simulink model "flyball"  (R2016b)
settings: Solver=VariableStepAuto  StartTime=0.0  StopTime=30  MaxStep=0.001  RelTol=1e-3
values from neighbouring files (symbols this model uses):
  g = 9.81    [simulateflyball.m]
  L = 0.2    [simulateflyball.m]
  M = 0.1    [simulateflyball.m]
  m = 0.2    [simulateflyball.m]
  thetaDotInitial = 0    [simulateflyball.m]
  thetaInitial = 0.0001    [simulateflyball.m]
  w = 6*pi    (= 18.8495559215)    [simulateflyball.m]
settings Model: Creator=kargto  LastModifiedBy=kargto

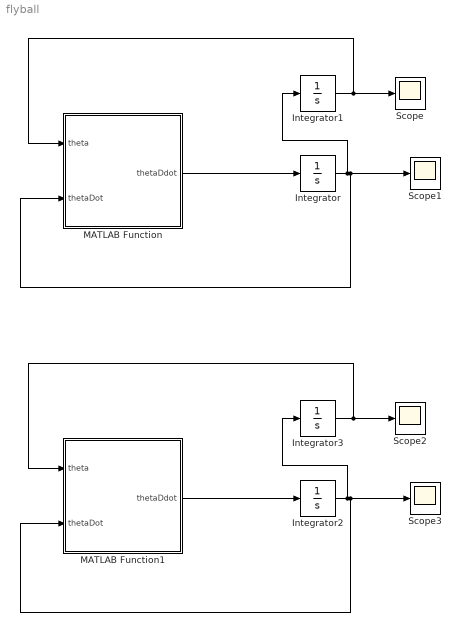
== system flyball ==
  Integrator : Integrator  InitialCondition=thetaDotInitial
  Integrator1 : Integrator  InitialCondition=thetaInitial
  Integrator2 : Integrator  InitialCondition=thetaDotInitial
  Integrator3 : Integrator  InitialCondition=thetaInitial
  MATLAB Function : MATLAB Function  TreatAsAtomicUnit=on
  MATLAB Function1 : MATLAB Function  TreatAsAtomicUnit=on
  Scope{,1..3} (4 alike) : Scope
  wires:
  MATLAB Function/1(thetaDdot) -> Integrator/1
  Integrator/1 -> Scope1/1, MATLAB Function/2(thetaDot), Integrator1/1
  Integrator1/1 -> MATLAB Function/1(theta), Scope/1
  MATLAB Function1/1(thetaDdot) -> Integrator2/1
  Integrator2/1 -> Integrator3/1, MATLAB Function1/2(thetaDot), Scope3/1
  Integrator3/1 -> Scope2/1, MATLAB Function1/1(theta)

== matlab function flyball/MATLAB Function1 ==
  data: theta input; thetaDdot output; thetaDot input; m parameter; M parameter; g parameter; L parameter; w parameter
function thetaDdot = fcn(theta,thetaDot,m, M, g, L, w)

thetaDdot = (sin(2*theta) * ( m*w^2/2) - g*sin(theta)*(m+M)/L)/(m+2*M*sin(theta)^2);

== matlab function flyball/MATLAB Function ==
  data: theta input; thetaDdot output; thetaDot input; m parameter; M parameter; g parameter; L parameter; w parameter
function thetaDdot = fcn(theta,thetaDot,m, M, g, L, w)

thetaDdot = (sin(2*theta) * ( m*w^2/2 - M*thetaDot) - g*sin(theta)*(m+M)/L)/(m+2*M*sin(theta)^2);
